simulink model "queue"  (R2024b)
settings: Solver=VariableStepAuto  StartTime=0.0  StopTime=100  RelTol=1e-3
undefined symbols (not defined in the file): m, n
settings Model: Creator=Botló  LastModifiedBy=Botló

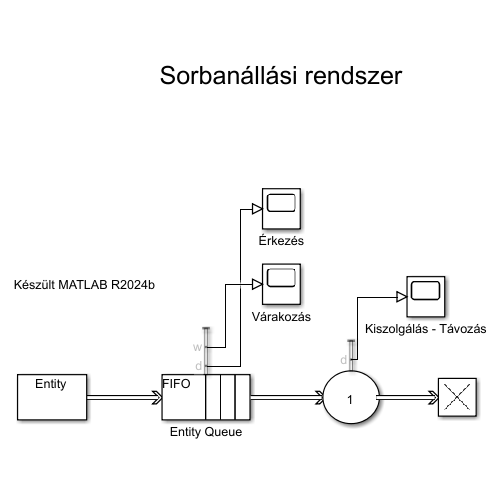
[thumbnail: Simulink's stored preview of the top-level diagram]
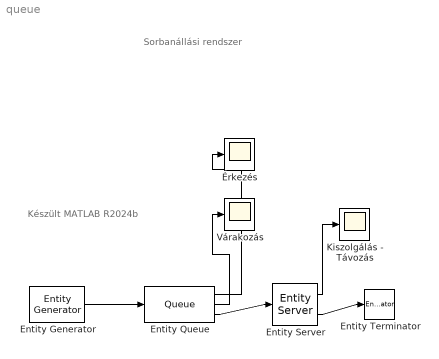
== system queue ==
  note: Készült MATLAB R2024b
  note: Sorbanállási rendszer
  Entity Generator : EntityGenerator  OutputPortMessageModes=m  EntityType=Structured  EntityTypeName=Entity
  Entity Queue : Queue  InputPortMessageModes=m  OutputPortMessageModes=n,n,m  Capacity=5  NumberEntitiesDeparted=on  AverageWait=on
      settings: OutputPortMap=o0,o2,o5
  Entity Server : EntityServer  InputPortMessageModes=m  OutputPortMessageModes=n,m  Capacity=1  ServiceTimeValue=5  NumberEntitiesDeparted=on
      settings: OutputPortMap=o0,o9
  Entity Terminator : EntityTerminator  InputPortMessageModes=m
  Kiszolgálás - Távozás : Scope
  Várakozás : Scope
  Érkezés : Scope
  wires:
  Entity Queue/3 -> Entity Server/1
  Entity Generator/1 -> Entity Queue/1
  Entity Server/1 -> Kiszolgálás - Távozás/1
  Entity Server/2 -> Entity Terminator/1
  Entity Queue/2 -> Várakozás/1
  Entity Queue/1 -> Érkezés/1
